simulink model "coalesce_walk_2d_sim"  (R2014b)
settings: Solver=ode45  StartTime=0.0  StopTime=t_end
InitFcn:
  | colors
  | simulation_params
  | mechanical_params
StartFcn:
  | tic
StopFcn:
  | stopscript
values from neighbouring files (symbols this model uses):
  b_hmotor = 0    [mechanical_params.m]
  b_leg_spring = 0.075*sqrt(k_leg_spring*0.5*.25^2)    [mechanical_params.m]
  b_rotor = 0*60/(2*pi)*9.725e-5    (= 0)    [mechanical_params.m]
  breakaway_friction = [25 25 25 25]    [mechanical_params.m]
  coulomb_friction = [20 20 20 20]    [mechanical_params.m]
  d_com = (d_hip_com_to_torso_com*m_torso)/(m_torso + num_legs*m_hshaft)    [mechanical_params.m]
  delta_phi_max = 160*pi/180    (= 2.79252680319)    [mechanical_params.m]
  delta_phi_min = 25.5*pi/180    (= 0.445058959259)    [mechanical_params.m]
  friction_linear_zone = [0.5 0.5 0.5 0.5].*pi/180    [mechanical_params.m]
  g = 9.81    [mechanical_params.m]
  HIP_MTR_MAX_TORQUE = max_current_hip*Kt_hip*N_h    (= 629.28)    [mechanical_params.m]
  initial_boom_pitch = 0    [mechanical_params.m]
  initial_boom_roll = asin((initial_com_height + boom_mount_to_com + boom_mount_to_center*tan(pitch_mount_angle) - (base_12(2) + yshaft_12(2))) / (l_boom + boom_mount_to_center_diagonal))    [mechanical_params.m]
  initial_boom_yaw = 0    [mechanical_params.m]
  initial_hip_roll = 0*pi/180    (= 0)    [mechanical_params.m]
  initial_winch_angle = -12 * pi/180    (= -0.209439510239)    [mechanical_params.m]
  k_gx = m_total*g/0.01    (= 57082.15332)    [mechanical_params.m]
  k_gy = m_total*g/0.005    (= 114164.30664)    [mechanical_params.m]
  k_leg_spring = 2950    [mechanical_params.m]
  k_phi = 5000    [mechanical_params.m]
  Kb_leg = 0.121    [mechanical_params.m]
  kd_winch = td_winch*kp_winch    (= 989.945961256)    [mechanical_params.m]
  kp_winch = winch_gravity_comp/(3*pi/180)    (= 19798.9192251)    [mechanical_params.m]
  Kt_leg = 0.121    [mechanical_params.m]
  L_leg = 0.102e-3    (= 0.000102)    [mechanical_params.m]
  l_seg = 0.5    [mechanical_params.m]
  LEG_MTR_MAX_TORQUE = max_current_leg * Kt_leg * N    (= 1210)    [mechanical_params.m]
  lowerleg_12 = 0.40    (= 0.4)    [mechanical_params.m]
  m_boom = 4.49    [mechanical_params.m]
  m_fblink = 0.46    [mechanical_params.m]
  m_hshaft = 18    [mechanical_params.m]
  m_lowerleg = 0.4438    [mechanical_params.m]
  m_output_gear = 1e-5    (= 1e-05)    [mechanical_params.m]
  m_rotor = 1e-5    (= 1e-05)    [mechanical_params.m]
  m_shin = 0.75    [mechanical_params.m]
  m_thigh = 0.69    [mechanical_params.m]
  m_torso = 17.5    [mechanical_params.m]
  m_total = num_legs*(m_hshaft + m_thigh + m_lowerleg + m_shin + m_fblink + 2*m_gearing) + m_torso    (= 58.18772)    [mechanical_params.m]
  m_virtual_gear = 1e-5    (= 1e-05)    [mechanical_params.m]
  m_yshaft = 12.89    [mechanical_params.m]
  max_current_leg = 200    [mechanical_params.m]
  max_voltage_leg = 50    [mechanical_params.m]
  mu_hmotor = 0.90    (= 0.9)    [mechanical_params.m]
  mu_motor = 0.85    [mechanical_params.m]
  mu_slide = 0.95    [mechanical_params.m]
  mu_stick = 1.00    (= 1)    [mechanical_params.m]
  N = 50    [mechanical_params.m]
  N_h = r_hip_shaft / r_hip_gearhead    (= 57)    [mechanical_params.m]
  phi_max_collision = -5*pi/180    (= -0.0872664625997)    [mechanical_params.m]
  phi_roll_max = pi + 16*pi/180    (= 3.42084533391)    [mechanical_params.m]
  phi_roll_min = pi - 9*pi/180    (= 2.98451302091)    [mechanical_params.m]
  phi_shin_max = 3*pi/2 + 17.5*pi/180    (= 5.01782159948)    [mechanical_params.m]
  phi_shin_min = pi - 45*pi/180    (= 2.35619449019)    [mechanical_params.m]
  phi_thigh_max = pi + 45*pi/180    (= 3.92699081699)    [mechanical_params.m]
  phi_thigh_min = pi/2 - 17.5*pi/180    (= 1.2653637077)    [mechanical_params.m]
  r_hip_gearhead = 0.009525    [mechanical_params.m]
  r_hip_shaft = 0.542925    [mechanical_params.m]
  R_leg = 0.052    [mechanical_params.m]
  r_rotor = 0.001    [mechanical_params.m]
  r_virtual_gear = N*r_rotor    (= 0.05)    [mechanical_params.m]
  s = clamp(s, 0, 1)    [controller.m]
  shin_12 = 0.40    (= 0.4)    [mechanical_params.m]
  shin_initial_l = initial_l_leg_angle + acos(initial_l_leg_length)    [mechanical_params.m]
  shin_initial_r = initial_r_leg_angle + acos(initial_r_leg_length)    [mechanical_params.m]
  thigh_initial_l = initial_l_leg_angle - acos(initial_l_leg_length)    [mechanical_params.m]
  thigh_initial_r = initial_r_leg_angle - acos(initial_r_leg_length)    [mechanical_params.m]
  tile_color = cmap(floor((tile_scale/(max_floor_tile_height+eps))*length(cmap))+1,:)    [mechanical_params.m]
  tile_cross_section = [1.5 0.03; 1.5 0; 3 0; 3 0.03]    [mechanical_params.m]
  tile_delta = [0 1; 0 0; 0 0; 0 1]    [mechanical_params.m]
  tile_scale = zeros(12, 1)    [mechanical_params.m]
  v_gx_max = 0.03    [mechanical_params.m]
  v_gy_max = 0.03    [mechanical_params.m]
  v_phi_max = 1/60    (= 0.0166666666667)    [mechanical_params.m]
  viscous_friction = [0.001 0.001 0.001 0.001]    [mechanical_params.m]
  vLimit = 0.01    [mechanical_params.m]
undefined symbols (not defined in the file or in its folder): A_lpf_velocity, B1_lpf_velocity, B2_lpf_velocity, base_color_d, boom_color_d, fblink_color_d, floor_color_d, hshaft_color_d, lowerleg_color_d, output_sample_time, rad, sample_time, sgn, shin_color_d, t_friction, thigh_color_d, torso_color_d, X, Y, yshaft_color_d, Z
libraries: sm_lib x196, nesl_utility x125, simulink x48, fl_lib x16, simulink_extras x2, mblibv1 x2, commnoisgen2 x1
(part 6 of 8)

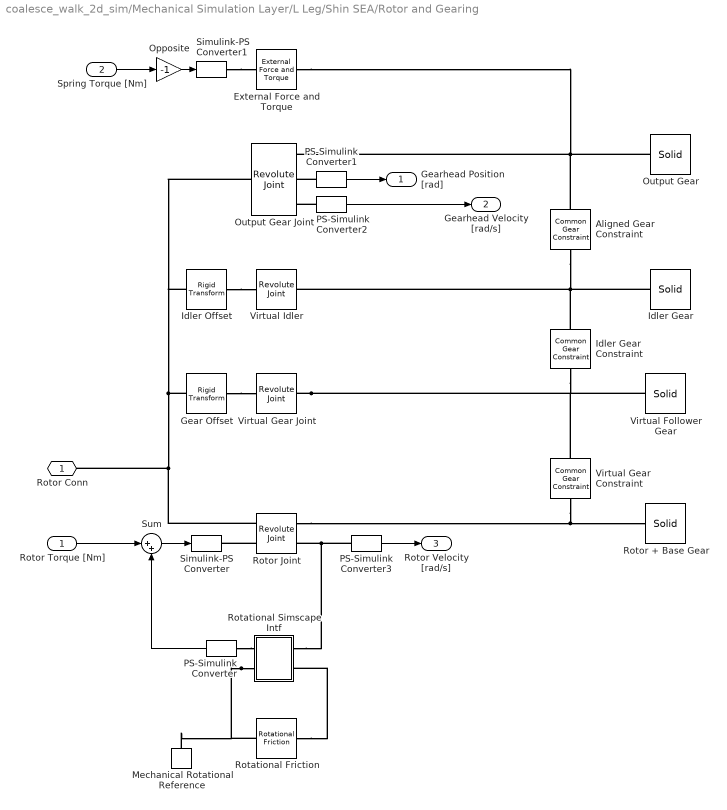
== system coalesce_walk_2d_sim/Mechanical Simulation Layer/L Leg/Shin SEA/Rotor and Gearing ==
  Rotor Torque [Nm] : Inport
  Spring Torque [Nm] : Inport  Port=2
  Aligned Gear Constraint : sm_lib/Gears and Couplings/Gears/Common Gear Constraint  GearType=External  SpecificationType=CenterDistanceRatio  CenterDistance=(r_rotor+r_virtual_gear)/2  CenterDistanceUnits=m  GearRatio=1  BaseGearRadius=1  BaseGearRadiusUnits=m  FollGearRadius=1  FollGearRadiusUnits=m  AssemblyGearRotation=Free  BlockFunction=simmechanics.library.gears_couplings_drives.gears.common_gear
  External Force and Torque : sm_lib/Forces and Torques/External Force and Torque  ForceResolutionFrame=AttachedFrame  EnableForceX=off  EnableForceY=off  EnableForceZ=off  EnableForce=off  TorqueResolutionFrame=AttachedFrame  EnableTorqueX=off  EnableTorqueY=off  EnableTorqueZ=on  EnableTorque=off  BlockFunction=simmechanics.library.forces_torques.external_force_torque
  Gear Offset : sm_lib/Frames and Transforms/Rigid Transform  TranslationMethod=Cartesian  TranslationLengthUnit=m  TranslationStandardAxis=+Z  TranslationStandardOffset=0  TranslationCartesianOffset=[(r_rotor+r_virtual_gear) 0 0]  TranslationROffset=0  TranslationROffsetUnits=m  TranslationZOffset=0  TranslationZOffsetUnits=m  TranslationThetaOffset=0  TranslationThetaOffsetUnits=deg  RotationMethod=None  RotationAngleUnits=deg  RotationStandardAxis=+Z  RotationAngle=0  RotationArbitraryAxis=[0 0 1]  FollAlignAxisA=+X  BaseAlignAxisA=+Y  FollAlignAxisB=+Y  BaseAlignAxisB=+Z  RotationMatrix=[1 0 0; 0 1 0; 0 0 1]  BlockFunction=simmechanics.library.frames_transforms.rigid_transform
  Idler Gear : sm_lib/Body Elements/Solid  InertiaType=Custom  Mass=m_virtual_gear  MassUnits=kg  CenterOfMass=[0 0 0]  CenterOfMassUnits=m  MomentsOfInertia=i_virtual_gear  MomentsOfInertiaUnits=kg*m^2  ProductsOfInertia=[0 0 0]  ProductsOfInertiaUnits=kg*m^2  DensityBased=on  Density=1000  DensityUnits=kg/(m^3)  GraphicType=None  MarkerShape=Sphere  MarkerSize=10  MarkerSizeUnits=m  GraphicVisPropType=SimpleVisualProperties  GraphicDiffuseColor=[1.0 0.2 0.2]  GraphicSpecularColor=[0.5 0.5 0.5 1.0]  GraphicAmbientColor=[0.15 0.15 0.15 1.0]  GraphicEmissiveColor=[0.0 0.0 0.0 1.0]  GraphicShininess=75  GraphicOpacity=1.0  GeometryShape=Cylinder  RectangleSize=[1 1]  RectangleSizeUnits=m  BrickDimensions=[1 1 1]  BrickDimensionUnits=m  CylinderRadius=r_virtual_gear  CylinderRadiusUnits=m  CylinderLength=0.01  CylinderLengthUnits=m  SphereRadius=1  SphereRadiusUnits=m  EllipsoidRadii=[1 1 1]  EllipsoidRadiiUnits=m  ExtrusionCrossSection=[1 1; -1 1; -1 -1; 1 -1]  ExtrusionCrossSectionUnits=m  ExtrusionLength=.2  ExtrusionLengthUnits=m  PolygonNumSides=3  PolygonOuterRadius=.3  PolygonOuterRadiusUnits=m  ExtGeomFileType=STL  ExtGeomFileUnits=m  RevolutionCrossSection=[1 1; 1 -1; 2 -1; 2 1]  RevolutionCrossSectionUnits=m  RevolutionExtent=Full  RevolutionAngle=180  RevolutionAngleUnits=deg  BlockFunction=simmechanics.library.body_elements.solid
  Idler Gear Constraint : sm_lib/Gears and Couplings/Gears/Common Gear Constraint  GearType=External  SpecificationType=CenterDistanceRatio  CenterDistance=(r_rotor+r_virtual_gear)/2  CenterDistanceUnits=m  GearRatio=1.0  BaseGearRadius=r_rotor  BaseGearRadiusUnits=m  FollGearRadius=r_virtual_gear  FollGearRadiusUnits=m  AssemblyGearRotation=Free  BlockFunction=simmechanics.library.gears_couplings_drives.gears.common_gear
  Idler Offset : sm_lib/Frames and Transforms/Rigid Transform  TranslationMethod=Cartesian  TranslationLengthUnit=m  TranslationStandardAxis=+Z  TranslationStandardOffset=0  TranslationCartesianOffset=[(r_rotor+r_virtual_gear)/2 0 0]  TranslationROffset=0  TranslationROffsetUnits=m  TranslationZOffset=0  TranslationZOffsetUnits=m  TranslationThetaOffset=0  TranslationThetaOffsetUnits=deg  RotationMethod=None  RotationAngleUnits=deg  RotationStandardAxis=+Z  RotationAngle=0  RotationArbitraryAxis=[0 0 1]  FollAlignAxisA=+X  BaseAlignAxisA=+Y  FollAlignAxisB=+Y  BaseAlignAxisB=+Z  RotationMatrix=[1 0 0; 0 1 0; 0 0 1]  BlockFunction=simmechanics.library.frames_transforms.rigid_transform
  Mechanical Rotational Reference : fl_lib/Mechanical/Rotational Elements/Mechanical Rotational Reference
  Opposite : Gain  Gain=-1
  Output Gear Joint : sm_lib/Joints/Revolute Joint  SenseConstraintForce=off  SenseConstraintForceX=off  SenseConstraintForceY=off  SenseConstraintForceZ=off  SenseConstraintTorque=off  SenseConstraintTorqueX=off  SenseConstraintTorqueY=off  SenseConstraintTorqueZ=off  SenseTotalForce=off  SenseTotalForceX=off  SenseTotalForceY=off  SenseTotalForceZ=off  SenseTotalTorque=off  SenseTotalTorqueX=off  SenseTotalTorqueY=off  SenseTotalTorqueZ=off  CompositeWrenchDir=FollowerOnBase  CompositeWrenchFrame=BaseFrame  EquilibriumPosition=0  EquilibriumPositionUnits=deg  SpringStiffness=0  SpringStiffnessUnits=N*m/deg  DampingCoefficient=0  DampingCoefficientUnits=N*m/(deg/s)  TorqueActuationMode=NoTorque  MotionActuationMode=ComputedMotion  SensePosition=on  SenseVelocity=on  SenseAcceleration=off  SenseTorqueForce=off  PositionTargetValue=0  PositionTargetValueUnits=deg  PositionTargetSpecify=off  PositionTargetPriority=High  VelocityTargetValue=0  VelocityTargetValueUnits=deg/s  VelocityTargetSpecify=off  VelocityTargetPriority=High  BlockFunction=simmechanics.library.joints.revolute_joint
  Output Gear : sm_lib/Body Elements/Solid  InertiaType=Custom  Mass=m_output_gear  MassUnits=kg  CenterOfMass=[0 0 0]  CenterOfMassUnits=m  MomentsOfInertia=i_output_gear  MomentsOfInertiaUnits=kg*m^2  ProductsOfInertia=[0 0 0]  ProductsOfInertiaUnits=kg*m^2  DensityBased=on  Density=1000  DensityUnits=kg/(m^3)  GraphicType=None  MarkerShape=Sphere  MarkerSize=10  MarkerSizeUnits=m  GraphicVisPropType=SimpleVisualProperties  GraphicDiffuseColor=[1.0 0.2 0.0]  GraphicSpecularColor=[0.5 0.5 0.5 1.0]  GraphicAmbientColor=[0.15 0.15 0.15 1.0]  GraphicEmissiveColor=[0.0 0.0 0.0 1.0]  GraphicShininess=75  GraphicOpacity=1.0  GeometryShape=Cylinder  RectangleSize=[1 1]  RectangleSizeUnits=m  BrickDimensions=[1 1 1]  BrickDimensionUnits=m  CylinderRadius=0.03  CylinderRadiusUnits=m  CylinderLength=0.01  CylinderLengthUnits=m  SphereRadius=1  SphereRadiusUnits=m  EllipsoidRadii=[1 1 1]  EllipsoidRadiiUnits=m  ExtrusionCrossSection=[1 1; -1 1; -1 -1; 1 -1]  ExtrusionCrossSectionUnits=m  ExtrusionLength=1  ExtrusionLengthUnits=m  PolygonNumSides=3  PolygonOuterRadius=1  PolygonOuterRadiusUnits=m  ExtGeomFileType=STL  ExtGeomFileUnits=m  RevolutionCrossSection=[1 1; 1 -1; 2 -1; 2 1]  RevolutionCrossSectionUnits=m  RevolutionExtent=Full  RevolutionAngle=180  RevolutionAngleUnits=deg  BlockFunction=simmechanics.library.body_elements.solid
  PS-Simulink Converter{,1..3} (4 alike) : nesl_utility/PS-Simulink Converter  PhysicalDomain=network_engine_domain  SubClassName=ps_output  LeftPortType=input  RightPortType=output  PseudoPeriodic=off  Frequencies=[]  Unit=1  AffineConversion=off
  Rotational Simscape Intf : Subsystem
  Rotational Friction : fl_lib/Mechanical/Rotational Elements/Rotational Friction  brkwy_trq=breakaway_friction(3)/N N*m  Col_trq=coulomb_friction(3)/N N*m  visc_coef=viscous_friction(3)/N N*m/(rad/s)  trans_coef=10 s/rad  vel_thr=friction_linear_zone(3)*N rad/s  w_specify=off  w_priority=High  w=0 rad/s  t_specify=off  t_priority=High  t=0 N*m
  Rotor + Base Gear : sm_lib/Body Elements/Solid  InertiaType=Custom  Mass=m_rotor  MassUnits=kg  CenterOfMass=[0 0 0]  CenterOfMassUnits=m  MomentsOfInertia=i_rotor_moments  MomentsOfInertiaUnits=kg*m^2  ProductsOfInertia=[0 0 0]  ProductsOfInertiaUnits=kg*m^2  DensityBased=on  Density=1000  DensityUnits=kg/(m^3)  GraphicType=None  MarkerShape=Sphere  MarkerSize=10  MarkerSizeUnits=m  GraphicVisPropType=AdvancedVisualProperties  GraphicDiffuseColor=[0.5 0.5 0.5]  GraphicSpecularColor=[0.5 0.5 0.5 1.0]  GraphicAmbientColor=[0.15 0.15 0.15 1.0]  GraphicEmissiveColor=[0.0 0.0 0.0 1.0]  GraphicShininess=10  GraphicOpacity=1.0  GeometryShape=Cylinder  RectangleSize=[1 1]  RectangleSizeUnits=m  BrickDimensions=[1 1 1]  BrickDimensionUnits=m  CylinderRadius=0.01  CylinderRadiusUnits=m  CylinderLength=0.01  CylinderLengthUnits=m  SphereRadius=1  SphereRadiusUnits=m  EllipsoidRadii=[1 1 1]  EllipsoidRadiiUnits=m  ExtrusionCrossSection=[1 1; -1 1; -1 -1; 1 -1]  ExtrusionCrossSectionUnits=m  ExtrusionLength=0.4  ExtrusionLengthUnits=m  PolygonNumSides=3  PolygonOuterRadius=0.2  PolygonOuterRadiusUnits=m  ExtGeomFileType=STL  ExtGeomFileUnits=m  RevolutionCrossSection=[1 1; 1 -1; 2 -1; 2 1]  RevolutionCrossSectionUnits=m  RevolutionExtent=Full  RevolutionAngle=180  RevolutionAngleUnits=deg  BlockFunction=simmechanics.library.body_elements.solid
  Rotor Joint : sm_lib/Joints/Revolute Joint  SenseConstraintForce=off  SenseConstraintForceX=off  SenseConstraintForceY=off  SenseConstraintForceZ=off  SenseConstraintTorque=off  SenseConstraintTorqueX=off  SenseConstraintTorqueY=off  SenseConstraintTorqueZ=off  SenseTotalForce=off  SenseTotalForceX=off  SenseTotalForceY=off  SenseTotalForceZ=off  SenseTotalTorque=off  SenseTotalTorqueX=off  SenseTotalTorqueY=off  SenseTotalTorqueZ=off  CompositeWrenchDir=FollowerOnBase  CompositeWrenchFrame=BaseFrame  EquilibriumPosition=0  EquilibriumPositionUnits=deg  SpringStiffness=0  SpringStiffnessUnits=N*m/deg  DampingCoefficient=0  DampingCoefficientUnits=N*m/(deg/s)  TorqueActuationMode=InputTorque  MotionActuationMode=ComputedMotion  SensePosition=off  SenseVelocity=on  SenseAcceleration=off  SenseTorqueForce=off  PositionTargetValue=0  PositionTargetValueUnits=deg  PositionTargetSpecify=off  PositionTargetPriority=High  VelocityTargetValue=0  VelocityTargetValueUnits=deg/s  VelocityTargetSpecify=off  VelocityTargetPriority=High  BlockFunction=simmechanics.library.joints.revolute_joint
  Simulink-PS Converter : nesl_utility/Simulink-PS Converter  PhysicalDomain=network_engine_domain  SubClassName=ps_input  LeftPortType=input  RightPortType=output  PseudoPeriodic=off  Frequencies=[]  NoiseDistribution=none  NoiseParameters=[]  Unit=1  AffineConversion=off  InputFiltering=off  SimscapeFilterOrder=1  InputFilterTimeConstant=0.001  UdotUserProvided=1
  Simulink-PS Converter1 : nesl_utility/Simulink-PS Converter  PhysicalDomain=network_engine_domain  SubClassName=ps_input  LeftPortType=input  RightPortType=output  PseudoPeriodic=off  Frequencies=[]  NoiseDistribution=none  NoiseParameters=[]  Unit=1  AffineConversion=off  InputFiltering=off  SimscapeFilterOrder=1  InputFilterTimeConstant=0.001  UdotUserProvided=1
  Sum : Sum  Inputs=|++
  Virtual Gear Joint : sm_lib/Joints/Revolute Joint  SenseConstraintForce=off  SenseConstraintForceX=off  SenseConstraintForceY=off  SenseConstraintForceZ=off  SenseConstraintTorque=off  SenseConstraintTorqueX=off  SenseConstraintTorqueY=off  SenseConstraintTorqueZ=off  SenseTotalForce=off  SenseTotalForceX=off  SenseTotalForceY=off  SenseTotalForceZ=off  SenseTotalTorque=off  SenseTotalTorqueX=off  SenseTotalTorqueY=off  SenseTotalTorqueZ=off  CompositeWrenchDir=FollowerOnBase  CompositeWrenchFrame=BaseFrame  EquilibriumPosition=0  EquilibriumPositionUnits=deg  SpringStiffness=0  SpringStiffnessUnits=N*m/deg  DampingCoefficient=0  DampingCoefficientUnits=N*m/(deg/s)  TorqueActuationMode=NoTorque  MotionActuationMode=ComputedMotion  SensePosition=off  SenseVelocity=off  SenseAcceleration=off  SenseTorqueForce=off  PositionTargetValue=0  PositionTargetValueUnits=deg  PositionTargetSpecify=off  PositionTargetPriority=High  VelocityTargetValue=0  VelocityTargetValueUnits=deg/s  VelocityTargetSpecify=off  VelocityTargetPriority=High  BlockFunction=simmechanics.library.joints.revolute_joint
  Virtual Follower Gear : sm_lib/Body Elements/Solid  InertiaType=Custom  Mass=m_virtual_gear  MassUnits=kg  CenterOfMass=[0 0 0]  CenterOfMassUnits=m  MomentsOfInertia=i_virtual_gear  MomentsOfInertiaUnits=kg*m^2  ProductsOfInertia=[0 0 0]  ProductsOfInertiaUnits=kg*m^2  DensityBased=on  Density=1000  DensityUnits=kg/(m^3)  GraphicType=None  MarkerShape=Sphere  MarkerSize=10  MarkerSizeUnits=m  GraphicVisPropType=SimpleVisualProperties  GraphicDiffuseColor=[1.0 0.2 0.2]  GraphicSpecularColor=[0.5 0.5 0.5 1.0]  GraphicAmbientColor=[0.15 0.15 0.15 1.0]  GraphicEmissiveColor=[0.0 0.0 0.0 1.0]  GraphicShininess=75  GraphicOpacity=1.0  GeometryShape=Cylinder  RectangleSize=[1 1]  RectangleSizeUnits=m  BrickDimensions=[1 1 1]  BrickDimensionUnits=m  CylinderRadius=r_virtual_gear  CylinderRadiusUnits=m  CylinderLength=0.01  CylinderLengthUnits=m  SphereRadius=1  SphereRadiusUnits=m  EllipsoidRadii=[1 1 1]  EllipsoidRadiiUnits=m  ExtrusionCrossSection=[1 1; -1 1; -1 -1; 1 -1]  ExtrusionCrossSectionUnits=m  ExtrusionLength=.2  ExtrusionLengthUnits=m  PolygonNumSides=3  PolygonOuterRadius=.3  PolygonOuterRadiusUnits=m  ExtGeomFileType=STL  ExtGeomFileUnits=m  RevolutionCrossSection=[1 1; 1 -1; 2 -1; 2 1]  RevolutionCrossSectionUnits=m  RevolutionExtent=Full  RevolutionAngle=180  RevolutionAngleUnits=deg  BlockFunction=simmechanics.library.body_elements.solid
  Virtual Gear Constraint : sm_lib/Gears and Couplings/Gears/Common Gear Constraint  GearType=External  SpecificationType=PitchCircleRadii  CenterDistance=20.0  CenterDistanceUnits=cm  GearRatio=1.0  BaseGearRadius=r_rotor  BaseGearRadiusUnits=m  FollGearRadius=r_virtual_gear  FollGearRadiusUnits=m  AssemblyGearRotation=Free  BlockFunction=simmechanics.library.gears_couplings_drives.gears.common_gear
  Virtual Idler : sm_lib/Joints/Revolute Joint  SenseConstraintForce=off  SenseConstraintForceX=off  SenseConstraintForceY=off  SenseConstraintForceZ=off  SenseConstraintTorque=off  SenseConstraintTorqueX=off  SenseConstraintTorqueY=off  SenseConstraintTorqueZ=off  SenseTotalForce=off  SenseTotalForceX=off  SenseTotalForceY=off  SenseTotalForceZ=off  SenseTotalTorque=off  SenseTotalTorqueX=off  SenseTotalTorqueY=off  SenseTotalTorqueZ=off  CompositeWrenchDir=FollowerOnBase  CompositeWrenchFrame=BaseFrame  EquilibriumPosition=0  EquilibriumPositionUnits=deg  SpringStiffness=0  SpringStiffnessUnits=N*m/deg  DampingCoefficient=0  DampingCoefficientUnits=N*m/(deg/s)  TorqueActuationMode=NoTorque  MotionActuationMode=ComputedMotion  SensePosition=off  SenseVelocity=off  SenseAcceleration=off  SenseTorqueForce=off  PositionTargetValue=0  PositionTargetValueUnits=deg  PositionTargetSpecify=off  PositionTargetPriority=High  VelocityTargetValue=0  VelocityTargetValueUnits=deg/s  VelocityTargetSpecify=off  VelocityTargetPriority=High  BlockFunction=simmechanics.library.joints.revolute_joint
  Rotor Conn : PMIOPort  Port=1  Side=Left
  Gearhead Position [rad] : Outport
  Gearhead Velocity [rad/s] : Outport  Port=2
  Rotor Velocity [rad/s] : Outport  Port=3
  wires:
  PS-Simulink Converter1/1 -> Gearhead Position [rad]/1
  Rotor Torque [Nm]/1 -> Sum/1
  PS-Simulink Converter2/1 -> Gearhead Velocity [rad/s]/1
  PS-Simulink Converter3/1 -> Rotor Velocity [rad/s]/1
  Spring Torque [Nm]/1 -> Opposite/1
  Opposite/1 -> Simulink-PS Converter1/1
  PS-Simulink Converter/1 -> Sum/2
  Sum/1 -> Simulink-PS Converter/1
  connections:
  Virtual Gear Joint/RConn1 -- Virtual Follower Gear/RConn1 -- Virtual Gear Constraint/RConn1 -- Idler Gear Constraint/LConn1
  External Force and Torque/RConn1 -- Output Gear/RConn1 -- Aligned Gear Constraint/RConn1 -- Output Gear Joint/RConn1
  Gear Offset/RConn1 -- Virtual Gear Joint/LConn1
  Gear Offset/LConn1 -- Rotor Joint/LConn1 -- Rotor Conn/RConn1 -- Output Gear Joint/LConn1 -- Idler Offset/LConn1
  Rotor Joint/RConn1 -- Virtual Gear Constraint/LConn1 -- Rotor + Base Gear/RConn1
  Rotor Joint/LConn2 -- Simulink-PS Converter/RConn1
  PS-Simulink Converter2/LConn1 -- Output Gear Joint/RConn3
  PS-Simulink Converter1/LConn1 -- Output Gear Joint/RConn2
  PS-Simulink Converter3/LConn1 -- Rotational Simscape Intf/LConn1 -- Rotor Joint/RConn2
  Simulink-PS Converter1/RConn1 -- External Force and Torque/LConn1
  Idler Gear Constraint/RConn1 -- Virtual Idler/RConn1 -- Idler Gear/RConn1 -- Aligned Gear Constraint/LConn1
  Idler Offset/RConn1 -- Virtual Idler/LConn1
  Rotational Simscape Intf/RConn2 -- Mechanical Rotational Reference/LConn1 -- Rotational Friction/RConn1
  Rotational Friction/LConn1 -- Rotational Simscape Intf/LConn2
  PS-Simulink Converter/LConn1 -- Rotational Simscape Intf/RConn1

== system coalesce_walk_2d_sim/Mechanical Simulation Layer/L Leg/Thigh/Frame Data ==
  Kinematic Data : ToWorkspace  VariableName=l_thigh_out  SampleTime=output_sample_time
      settings: Save2DSignal=2-D array (concatenate along first dimension)
  Mux : Mux
  PS-Simulink Converter{,1..3} (4 alike) : nesl_utility/PS-Simulink Converter  PhysicalDomain=network_engine_domain  SubClassName=ps_output  LeftPortType=input  RightPortType=output  PseudoPeriodic=off  Frequencies=[]  Unit=1  AffineConversion=off
  Transform Sensor : sm_lib/Frames and Transforms/Transform Sensor  MeasurementFrame=World  SenseAngle=off  SenseAxis=off  SenseAngle1=off  SenseAngle2=off  SenseAngle3=off  SenseQ=on  SenseR=off  SenseOmegaX=off  SenseOmegaY=off  SenseOmegaZ=off  SenseOmega1=off  SenseOmega2=off  SenseOmega3=off  SenseQDot=off  SenseRDot=off  SenseAlphaX=off  SenseAlphaY=off  SenseAlphaZ=off  SenseAlpha1=off  SenseAlpha2=off  SenseAlpha3=off  SenseQDDot=off  SenseRDDot=off  SenseX=on  SenseY=on  SenseZ=on  SenseRad=off  SenseAzim=off  SenseDist=off  SenseInc=off  SenseXDot=off  SenseYDot=off  SenseZDot=off  SenseRadDot=off  SenseAzimDot=off  SenseDistDot=off  SenseIncDot=off  SenseXDDot=off  SenseYDDot=off  SenseZDDot=off  SenseRadDDot=off  SenseAzimDDot=off  SenseDistDDot=off  SenseIncDDot=off  BlockFunction=simmechanics.library.frames_transforms.transform_sensor
  World Frame : sm_lib/Frames and Transforms/World Frame  BlockFunction=simmechanics.library.frames_transforms.world_frame
  Frame : PMIOPort  Port=1  Side=Left
  wires:
  Mux/1 -> Kinematic Data/1
  PS-Simulink Converter/1 -> Mux/1
  PS-Simulink Converter1/1 -> Mux/2
  PS-Simulink Converter2/1 -> Mux/3
  PS-Simulink Converter3/1 -> Mux/4
  connections:
  PS-Simulink Converter3/LConn1 -- Transform Sensor/RConn5
  PS-Simulink Converter2/LConn1 -- Transform Sensor/RConn4
  PS-Simulink Converter1/LConn1 -- Transform Sensor/RConn3
  PS-Simulink Converter/LConn1 -- Transform Sensor/RConn2
  Transform Sensor/RConn1 -- Frame/RConn1
  Transform Sensor/LConn1 -- World Frame/RConn1

== system coalesce_walk_2d_sim/Mechanical Simulation Layer/L Leg/Thigh SEA/Motor Controller ==
  Desired Current [A] : Inport
  Measured Current [A] : Inport  Port=2
  Speed [rad/s] : Inport  Port=3
  Ke : Gain  Gain=Kb_leg
  PI Controller : simulink/Continuous/PID Controller  Controller=PI  TimeDomain=Continuous-time  SampleTime=-1  IntegratorMethod=Trapezoidal  FilterMethod=Forward Euler  Form=Parallel  P=0.57  I=0.016  D=0.016  N=10  InitialConditionSource=internal  InitialConditionForIntegrator=0  InitialConditionForFilter=0  ExternalReset=none  ZeroCross=off  LimitOutput=off  UpperSaturationLimit=inf  LowerSaturationLimit=-inf  LinearizeAsGain=on  AntiWindupMode=none  Kb=1  TrackingMode=off  Kt=1  PParamMin=[]  PParamMax=[]  IParamMin=[]  IParamMax=[]  DParamMin=[]  DParamMax=[]  NParamMin=[]  NParamMax=[]  KbParamMin=[]  KbParamMax=[]  KtParamMin=[]  KtParamMax=[]  POutMin=[]  POutMax=[]  IOutMin=[]  IOutMax=[]  DOutMin=[]  DOutMax=[]  NOutMin=[]  NOutMax=[]  KbOutMin=[]  KbOutMax=[]  KtOutMin=[]  KtOutMax=[]  IntegratorOutMin=[]  IntegratorOutMax=[]  FilterOutMin=[]  FilterOutMax=[]  SumOutMin=[]  SumOutMax=[]  SumI1OutMin=[]  SumI1OutMax=[]  SumI2OutMin=[]  SumI2OutMax=[]  SumI3OutMin=[]  SumI3OutMax=[]  SumDOutMin=[]  SumDOutMax=[]  SaturationOutMin=[]  SaturationOutMax=[]  IntegratorContinuousStateAttributes=''  IntegratorStateMustResolveToSignalObject=off  IntegratorRTWStateStorageClass=Auto  FilterContinuousStateAttributes=''  FilterStateMustResolveToSignalObject=off  FilterRTWStateStorageClass=Auto  DifferentiatorICPrevScaledInput=0  DifferentiatorOutMin=[]  DifferentiatorOutMax=[]  UseFilter=on
  Resistance : Gain  Gain=R_leg
  Sum : Sum  Inputs=|+-
  Sum1 : Sum  Inputs=|++
  Sum2 : Sum  Inputs=+|+
  Voltage [V] : Outport
  wires:
  Desired Current [A]/1 -> Sum/1
  Measured Current [A]/1 -> Resistance/1, Sum/2
  Sum/1 -> PI Controller/1
  PI Controller/1 -> Sum1/1
  Speed [rad/s]/1 -> Ke/1
  Sum2/1 -> Sum1/2
  Resistance/1 -> Sum2/1
  Ke/1 -> Sum2/2
  Sum1/1 -> Voltage [V]/1

== system coalesce_walk_2d_sim/Mechanical Simulation Layer/L Leg/Thigh SEA/Motor Electromagnetism ==
  Voltage [V] : Inport
  Speed [rad/s] : Inport  Port=2
  Add : Sum  Inputs=-+-
  Inductance : Gain  Gain=1/L_leg
  Integrator : Integrator  ZeroCross=off
  Ke : Gain  Gain=Kb_leg
  Resistance : Gain  Gain=R_leg
  Torque Limiter (outside) 1 : Saturate  UpperLimit=max_voltage_leg  LowerLimit=-max_voltage_leg  ZeroCross=off
      settings: AttributesFormatString=Hi: %<UpperLimit>\nLo: %<LowerLimit>
  Torque Limiter (outside) 2 : Saturate  UpperLimit=max_current_leg  LowerLimit=-max_current_leg  ZeroCross=off
      settings: AttributesFormatString=Hi: %<UpperLimit>\nLo: %<LowerLimit>
  Current [A] : Outport
  wires:
  Integrator/1 -> Torque Limiter (outside) 2/1  "I"
  Inductance/1 -> Integrator/1  "d/dt(I)"
  Speed [rad/s]/1 -> Ke/1  "d/dt(theta)"
  Add/1 -> Inductance/1
  Resistance/1 -> Add/1
  Ke/1 -> Add/3
  Voltage [V]/1 -> Torque Limiter (outside) 1/1
  Torque Limiter (outside) 2/1 -> Current [A]/1, Resistance/1
  Torque Limiter (outside) 1/1 -> Add/2

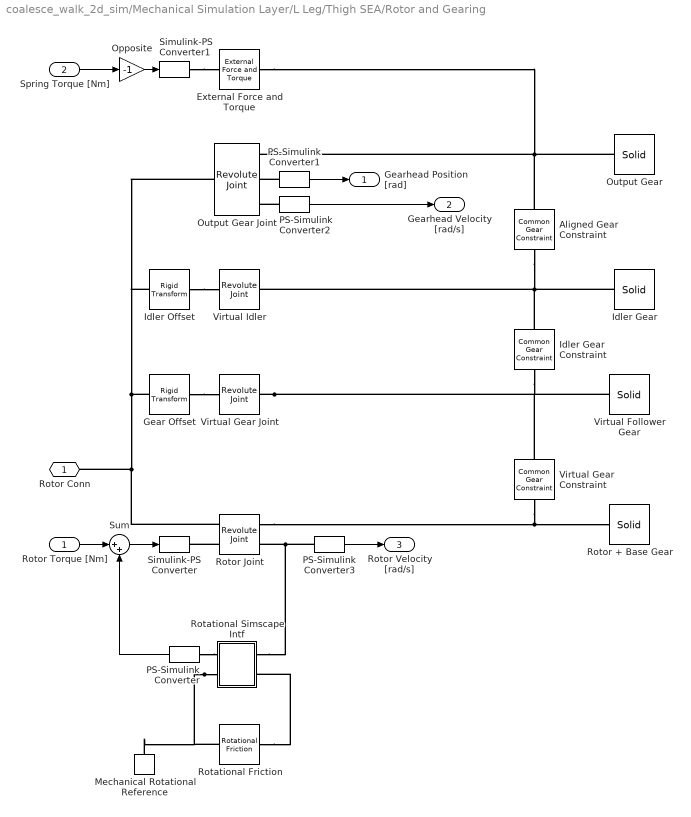
== system coalesce_walk_2d_sim/Mechanical Simulation Layer/L Leg/Thigh SEA/Rotor and Gearing ==
  Rotor Torque [Nm] : Inport
  Spring Torque [Nm] : Inport  Port=2
  Aligned Gear Constraint : sm_lib/Gears and Couplings/Gears/Common Gear Constraint  GearType=External  SpecificationType=CenterDistanceRatio  CenterDistance=(r_rotor+r_virtual_gear)/2  CenterDistanceUnits=m  GearRatio=1  BaseGearRadius=1  BaseGearRadiusUnits=m  FollGearRadius=1  FollGearRadiusUnits=m  AssemblyGearRotation=Free  BlockFunction=simmechanics.library.gears_couplings_drives.gears.common_gear
  External Force and Torque : sm_lib/Forces and Torques/External Force and Torque  ForceResolutionFrame=AttachedFrame  EnableForceX=off  EnableForceY=off  EnableForceZ=off  EnableForce=off  TorqueResolutionFrame=AttachedFrame  EnableTorqueX=off  EnableTorqueY=off  EnableTorqueZ=on  EnableTorque=off  BlockFunction=simmechanics.library.forces_torques.external_force_torque
  Gear Offset : sm_lib/Frames and Transforms/Rigid Transform  TranslationMethod=Cartesian  TranslationLengthUnit=m  TranslationStandardAxis=+Z  TranslationStandardOffset=0  TranslationCartesianOffset=[(r_rotor+r_virtual_gear) 0 0]  TranslationROffset=0  TranslationROffsetUnits=m  TranslationZOffset=0  TranslationZOffsetUnits=m  TranslationThetaOffset=0  TranslationThetaOffsetUnits=deg  RotationMethod=None  RotationAngleUnits=deg  RotationStandardAxis=+Z  RotationAngle=0  RotationArbitraryAxis=[0 0 1]  FollAlignAxisA=+X  BaseAlignAxisA=+Y  FollAlignAxisB=+Y  BaseAlignAxisB=+Z  RotationMatrix=[1 0 0; 0 1 0; 0 0 1]  BlockFunction=simmechanics.library.frames_transforms.rigid_transform
  Idler Gear : sm_lib/Body Elements/Solid  InertiaType=Custom  Mass=m_virtual_gear  MassUnits=kg  CenterOfMass=[0 0 0]  CenterOfMassUnits=m  MomentsOfInertia=i_virtual_gear  MomentsOfInertiaUnits=kg*m^2  ProductsOfInertia=[0 0 0]  ProductsOfInertiaUnits=kg*m^2  DensityBased=on  Density=1000  DensityUnits=kg/(m^3)  GraphicType=None  MarkerShape=Sphere  MarkerSize=10  MarkerSizeUnits=m  GraphicVisPropType=SimpleVisualProperties  GraphicDiffuseColor=[1.0 0.2 0.2]  GraphicSpecularColor=[0.5 0.5 0.5 1.0]  GraphicAmbientColor=[0.15 0.15 0.15 1.0]  GraphicEmissiveColor=[0.0 0.0 0.0 1.0]  GraphicShininess=75  GraphicOpacity=1.0  GeometryShape=Cylinder  RectangleSize=[1 1]  RectangleSizeUnits=m  BrickDimensions=[1 1 1]  BrickDimensionUnits=m  CylinderRadius=r_virtual_gear  CylinderRadiusUnits=m  CylinderLength=0.01  CylinderLengthUnits=m  SphereRadius=1  SphereRadiusUnits=m  EllipsoidRadii=[1 1 1]  EllipsoidRadiiUnits=m  ExtrusionCrossSection=[1 1; -1 1; -1 -1; 1 -1]  ExtrusionCrossSectionUnits=m  ExtrusionLength=.2  ExtrusionLengthUnits=m  PolygonNumSides=3  PolygonOuterRadius=.3  PolygonOuterRadiusUnits=m  ExtGeomFileType=STL  ExtGeomFileUnits=m  RevolutionCrossSection=[1 1; 1 -1; 2 -1; 2 1]  RevolutionCrossSectionUnits=m  RevolutionExtent=Full  RevolutionAngle=180  RevolutionAngleUnits=deg  BlockFunction=simmechanics.library.body_elements.solid
  Idler Gear Constraint : sm_lib/Gears and Couplings/Gears/Common Gear Constraint  GearType=External  SpecificationType=CenterDistanceRatio  CenterDistance=(r_rotor+r_virtual_gear)/2  CenterDistanceUnits=m  GearRatio=1.0  BaseGearRadius=r_rotor  BaseGearRadiusUnits=m  FollGearRadius=r_virtual_gear  FollGearRadiusUnits=m  AssemblyGearRotation=Free  BlockFunction=simmechanics.library.gears_couplings_drives.gears.common_gear
  Idler Offset : sm_lib/Frames and Transforms/Rigid Transform  TranslationMethod=Cartesian  TranslationLengthUnit=m  TranslationStandardAxis=+Z  TranslationStandardOffset=0  TranslationCartesianOffset=[(r_rotor+r_virtual_gear)/2 0 0]  TranslationROffset=0  TranslationROffsetUnits=m  TranslationZOffset=0  TranslationZOffsetUnits=m  TranslationThetaOffset=0  TranslationThetaOffsetUnits=deg  RotationMethod=None  RotationAngleUnits=deg  RotationStandardAxis=+Z  RotationAngle=0  RotationArbitraryAxis=[0 0 1]  FollAlignAxisA=+X  BaseAlignAxisA=+Y  FollAlignAxisB=+Y  BaseAlignAxisB=+Z  RotationMatrix=[1 0 0; 0 1 0; 0 0 1]  BlockFunction=simmechanics.library.frames_transforms.rigid_transform
  Mechanical Rotational Reference : fl_lib/Mechanical/Rotational Elements/Mechanical Rotational Reference
  Opposite : Gain  Gain=-1
  Output Gear Joint : sm_lib/Joints/Revolute Joint  SenseConstraintForce=off  SenseConstraintForceX=off  SenseConstraintForceY=off  SenseConstraintForceZ=off  SenseConstraintTorque=off  SenseConstraintTorqueX=off  SenseConstraintTorqueY=off  SenseConstraintTorqueZ=off  SenseTotalForce=off  SenseTotalForceX=off  SenseTotalForceY=off  SenseTotalForceZ=off  SenseTotalTorque=off  SenseTotalTorqueX=off  SenseTotalTorqueY=off  SenseTotalTorqueZ=off  CompositeWrenchDir=FollowerOnBase  CompositeWrenchFrame=BaseFrame  EquilibriumPosition=0  EquilibriumPositionUnits=deg  SpringStiffness=0  SpringStiffnessUnits=N*m/deg  DampingCoefficient=0  DampingCoefficientUnits=N*m/(deg/s)  TorqueActuationMode=NoTorque  MotionActuationMode=ComputedMotion  SensePosition=on  SenseVelocity=on  SenseAcceleration=off  SenseTorqueForce=off  PositionTargetValue=0  PositionTargetValueUnits=deg  PositionTargetSpecify=off  PositionTargetPriority=High  VelocityTargetValue=0  VelocityTargetValueUnits=deg/s  VelocityTargetSpecify=off  VelocityTargetPriority=High  BlockFunction=simmechanics.library.joints.revolute_joint
  Output Gear : sm_lib/Body Elements/Solid  InertiaType=Custom  Mass=m_output_gear  MassUnits=kg  CenterOfMass=[0 0 0]  CenterOfMassUnits=m  MomentsOfInertia=i_output_gear  MomentsOfInertiaUnits=kg*m^2  ProductsOfInertia=[0 0 0]  ProductsOfInertiaUnits=kg*m^2  DensityBased=on  Density=1000  DensityUnits=kg/(m^3)  GraphicType=None  MarkerShape=Sphere  MarkerSize=10  MarkerSizeUnits=m  GraphicVisPropType=SimpleVisualProperties  GraphicDiffuseColor=[1.0 0.2 0.0]  GraphicSpecularColor=[0.5 0.5 0.5 1.0]  GraphicAmbientColor=[0.15 0.15 0.15 1.0]  GraphicEmissiveColor=[0.0 0.0 0.0 1.0]  GraphicShininess=75  GraphicOpacity=1.0  GeometryShape=Cylinder  RectangleSize=[1 1]  RectangleSizeUnits=m  BrickDimensions=[1 1 1]  BrickDimensionUnits=m  CylinderRadius=0.03  CylinderRadiusUnits=m  CylinderLength=0.01  CylinderLengthUnits=m  SphereRadius=1  SphereRadiusUnits=m  EllipsoidRadii=[1 1 1]  EllipsoidRadiiUnits=m  ExtrusionCrossSection=[1 1; -1 1; -1 -1; 1 -1]  ExtrusionCrossSectionUnits=m  ExtrusionLength=1  ExtrusionLengthUnits=m  PolygonNumSides=3  PolygonOuterRadius=1  PolygonOuterRadiusUnits=m  ExtGeomFileType=STL  ExtGeomFileUnits=m  RevolutionCrossSection=[1 1; 1 -1; 2 -1; 2 1]  RevolutionCrossSectionUnits=m  RevolutionExtent=Full  RevolutionAngle=180  RevolutionAngleUnits=deg  BlockFunction=simmechanics.library.body_elements.solid
  PS-Simulink Converter{,1..3} (4 alike) : nesl_utility/PS-Simulink Converter  PhysicalDomain=network_engine_domain  SubClassName=ps_output  LeftPortType=input  RightPortType=output  PseudoPeriodic=off  Frequencies=[]  Unit=1  AffineConversion=off
  Rotational Simscape Intf : Subsystem
  Rotational Friction : fl_lib/Mechanical/Rotational Elements/Rotational Friction  brkwy_trq=breakaway_friction(4)/N N*m  Col_trq=coulomb_friction(4)/N N*m  visc_coef=viscous_friction(4)/N N*m/(rad/s)  trans_coef=10 s/rad  vel_thr=friction_linear_zone(4)*N rad/s  w_specify=off  w_priority=High  w=0 rad/s  t_specify=off  t_priority=High  t=0 N*m
  Rotor + Base Gear : sm_lib/Body Elements/Solid  InertiaType=Custom  Mass=m_rotor  MassUnits=kg  CenterOfMass=[0 0 0]  CenterOfMassUnits=m  MomentsOfInertia=i_rotor_moments  MomentsOfInertiaUnits=kg*m^2  ProductsOfInertia=[0 0 0]  ProductsOfInertiaUnits=kg*m^2  DensityBased=on  Density=1000  DensityUnits=kg/(m^3)  GraphicType=None  MarkerShape=Sphere  MarkerSize=10  MarkerSizeUnits=m  GraphicVisPropType=AdvancedVisualProperties  GraphicDiffuseColor=[0.5 0.5 0.5]  GraphicSpecularColor=[0.5 0.5 0.5 1.0]  GraphicAmbientColor=[0.15 0.15 0.15 1.0]  GraphicEmissiveColor=[0.0 0.0 0.0 1.0]  GraphicShininess=10  GraphicOpacity=1.0  GeometryShape=Cylinder  RectangleSize=[1 1]  RectangleSizeUnits=m  BrickDimensions=[1 1 1]  BrickDimensionUnits=m  CylinderRadius=0.01  CylinderRadiusUnits=m  CylinderLength=0.01  CylinderLengthUnits=m  SphereRadius=1  SphereRadiusUnits=m  EllipsoidRadii=[1 1 1]  EllipsoidRadiiUnits=m  ExtrusionCrossSection=[1 1; -1 1; -1 -1; 1 -1]  ExtrusionCrossSectionUnits=m  ExtrusionLength=0.4  ExtrusionLengthUnits=m  PolygonNumSides=3  PolygonOuterRadius=0.2  PolygonOuterRadiusUnits=m  ExtGeomFileType=STL  ExtGeomFileUnits=m  RevolutionCrossSection=[1 1; 1 -1; 2 -1; 2 1]  RevolutionCrossSectionUnits=m  RevolutionExtent=Full  RevolutionAngle=180  RevolutionAngleUnits=deg  BlockFunction=simmechanics.library.body_elements.solid
  Rotor Joint : sm_lib/Joints/Revolute Joint  SenseConstraintForce=off  SenseConstraintForceX=off  SenseConstraintForceY=off  SenseConstraintForceZ=off  SenseConstraintTorque=off  SenseConstraintTorqueX=off  SenseConstraintTorqueY=off  SenseConstraintTorqueZ=off  SenseTotalForce=off  SenseTotalForceX=off  SenseTotalForceY=off  SenseTotalForceZ=off  SenseTotalTorque=off  SenseTotalTorqueX=off  SenseTotalTorqueY=off  SenseTotalTorqueZ=off  CompositeWrenchDir=FollowerOnBase  CompositeWrenchFrame=BaseFrame  EquilibriumPosition=0  EquilibriumPositionUnits=deg  SpringStiffness=0  SpringStiffnessUnits=N*m/deg  DampingCoefficient=0  DampingCoefficientUnits=N*m/(deg/s)  TorqueActuationMode=InputTorque  MotionActuationMode=ComputedMotion  SensePosition=off  SenseVelocity=on  SenseAcceleration=off  SenseTorqueForce=off  PositionTargetValue=0  PositionTargetValueUnits=deg  PositionTargetSpecify=off  PositionTargetPriority=High  VelocityTargetValue=0  VelocityTargetValueUnits=deg/s  VelocityTargetSpecify=off  VelocityTargetPriority=High  BlockFunction=simmechanics.library.joints.revolute_joint
  Simulink-PS Converter : nesl_utility/Simulink-PS Converter  PhysicalDomain=network_engine_domain  SubClassName=ps_input  LeftPortType=input  RightPortType=output  PseudoPeriodic=off  Frequencies=[]  NoiseDistribution=none  NoiseParameters=[]  Unit=1  AffineConversion=off  InputFiltering=off  SimscapeFilterOrder=1  InputFilterTimeConstant=0.001  UdotUserProvided=1
  Simulink-PS Converter1 : nesl_utility/Simulink-PS Converter  PhysicalDomain=network_engine_domain  SubClassName=ps_input  LeftPortType=input  RightPortType=output  PseudoPeriodic=off  Frequencies=[]  NoiseDistribution=none  NoiseParameters=[]  Unit=1  AffineConversion=off  InputFiltering=off  SimscapeFilterOrder=1  InputFilterTimeConstant=0.001  UdotUserProvided=1
  Sum : Sum  Inputs=|++
  Virtual Gear Joint : sm_lib/Joints/Revolute Joint  SenseConstraintForce=off  SenseConstraintForceX=off  SenseConstraintForceY=off  SenseConstraintForceZ=off  SenseConstraintTorque=off  SenseConstraintTorqueX=off  SenseConstraintTorqueY=off  SenseConstraintTorqueZ=off  SenseTotalForce=off  SenseTotalForceX=off  SenseTotalForceY=off  SenseTotalForceZ=off  SenseTotalTorque=off  SenseTotalTorqueX=off  SenseTotalTorqueY=off  SenseTotalTorqueZ=off  CompositeWrenchDir=FollowerOnBase  CompositeWrenchFrame=BaseFrame  EquilibriumPosition=0  EquilibriumPositionUnits=deg  SpringStiffness=0  SpringStiffnessUnits=N*m/deg  DampingCoefficient=0  DampingCoefficientUnits=N*m/(deg/s)  TorqueActuationMode=NoTorque  MotionActuationMode=ComputedMotion  SensePosition=off  SenseVelocity=off  SenseAcceleration=off  SenseTorqueForce=off  PositionTargetValue=0  PositionTargetValueUnits=deg  PositionTargetSpecify=off  PositionTargetPriority=High  VelocityTargetValue=0  VelocityTargetValueUnits=deg/s  VelocityTargetSpecify=off  VelocityTargetPriority=High  BlockFunction=simmechanics.library.joints.revolute_joint
  Virtual Follower Gear : sm_lib/Body Elements/Solid  InertiaType=Custom  Mass=m_virtual_gear  MassUnits=kg  CenterOfMass=[0 0 0]  CenterOfMassUnits=m  MomentsOfInertia=i_virtual_gear  MomentsOfInertiaUnits=kg*m^2  ProductsOfInertia=[0 0 0]  ProductsOfInertiaUnits=kg*m^2  DensityBased=on  Density=1000  DensityUnits=kg/(m^3)  GraphicType=None  MarkerShape=Sphere  MarkerSize=10  MarkerSizeUnits=m  GraphicVisPropType=SimpleVisualProperties  GraphicDiffuseColor=[1.0 0.2 0.2]  GraphicSpecularColor=[0.5 0.5 0.5 1.0]  GraphicAmbientColor=[0.15 0.15 0.15 1.0]  GraphicEmissiveColor=[0.0 0.0 0.0 1.0]  GraphicShininess=75  GraphicOpacity=1.0  GeometryShape=Cylinder  RectangleSize=[1 1]  RectangleSizeUnits=m  BrickDimensions=[1 1 1]  BrickDimensionUnits=m  CylinderRadius=r_virtual_gear  CylinderRadiusUnits=m  CylinderLength=0.01  CylinderLengthUnits=m  SphereRadius=1  SphereRadiusUnits=m  EllipsoidRadii=[1 1 1]  EllipsoidRadiiUnits=m  ExtrusionCrossSection=[1 1; -1 1; -1 -1; 1 -1]  ExtrusionCrossSectionUnits=m  ExtrusionLength=.2  ExtrusionLengthUnits=m  PolygonNumSides=3  PolygonOuterRadius=.3  PolygonOuterRadiusUnits=m  ExtGeomFileType=STL  ExtGeomFileUnits=m  RevolutionCrossSection=[1 1; 1 -1; 2 -1; 2 1]  RevolutionCrossSectionUnits=m  RevolutionExtent=Full  RevolutionAngle=180  RevolutionAngleUnits=deg  BlockFunction=simmechanics.library.body_elements.solid
  Virtual Gear Constraint : sm_lib/Gears and Couplings/Gears/Common Gear Constraint  GearType=External  SpecificationType=PitchCircleRadii  CenterDistance=20.0  CenterDistanceUnits=cm  GearRatio=1.0  BaseGearRadius=r_rotor  BaseGearRadiusUnits=m  FollGearRadius=r_virtual_gear  FollGearRadiusUnits=m  AssemblyGearRotation=Free  BlockFunction=simmechanics.library.gears_couplings_drives.gears.common_gear
  Virtual Idler : sm_lib/Joints/Revolute Joint  SenseConstraintForce=off  SenseConstraintForceX=off  SenseConstraintForceY=off  SenseConstraintForceZ=off  SenseConstraintTorque=off  SenseConstraintTorqueX=off  SenseConstraintTorqueY=off  SenseConstraintTorqueZ=off  SenseTotalForce=off  SenseTotalForceX=off  SenseTotalForceY=off  SenseTotalForceZ=off  SenseTotalTorque=off  SenseTotalTorqueX=off  SenseTotalTorqueY=off  SenseTotalTorqueZ=off  CompositeWrenchDir=FollowerOnBase  CompositeWrenchFrame=BaseFrame  EquilibriumPosition=0  EquilibriumPositionUnits=deg  SpringStiffness=0  SpringStiffnessUnits=N*m/deg  DampingCoefficient=0  DampingCoefficientUnits=N*m/(deg/s)  TorqueActuationMode=NoTorque  MotionActuationMode=ComputedMotion  SensePosition=off  SenseVelocity=off  SenseAcceleration=off  SenseTorqueForce=off  PositionTargetValue=0  PositionTargetValueUnits=deg  PositionTargetSpecify=off  PositionTargetPriority=High  VelocityTargetValue=0  VelocityTargetValueUnits=deg/s  VelocityTargetSpecify=off  VelocityTargetPriority=High  BlockFunction=simmechanics.library.joints.revolute_joint
  Rotor Conn : PMIOPort  Port=1  Side=Left
  Gearhead Position [rad] : Outport
  Gearhead Velocity [rad/s] : Outport  Port=2
  Rotor Velocity [rad/s] : Outport  Port=3
  wires:
  PS-Simulink Converter1/1 -> Gearhead Position [rad]/1
  Rotor Torque [Nm]/1 -> Sum/1
  PS-Simulink Converter2/1 -> Gearhead Velocity [rad/s]/1
  PS-Simulink Converter3/1 -> Rotor Velocity [rad/s]/1
  Spring Torque [Nm]/1 -> Opposite/1
  Opposite/1 -> Simulink-PS Converter1/1
  PS-Simulink Converter/1 -> Sum/2
  Sum/1 -> Simulink-PS Converter/1
  connections:
  Virtual Gear Joint/RConn1 -- Virtual Follower Gear/RConn1 -- Virtual Gear Constraint/RConn1 -- Idler Gear Constraint/LConn1
  External Force and Torque/RConn1 -- Output Gear/RConn1 -- Aligned Gear Constraint/RConn1 -- Output Gear Joint/RConn1
  Gear Offset/RConn1 -- Virtual Gear Joint/LConn1
  Gear Offset/LConn1 -- Rotor Joint/LConn1 -- Rotor Conn/RConn1 -- Output Gear Joint/LConn1 -- Idler Offset/LConn1
  Rotor Joint/RConn1 -- Virtual Gear Constraint/LConn1 -- Rotor + Base Gear/RConn1
  Rotor Joint/LConn2 -- Simulink-PS Converter/RConn1
  PS-Simulink Converter2/LConn1 -- Output Gear Joint/RConn3
  PS-Simulink Converter1/LConn1 -- Output Gear Joint/RConn2
  PS-Simulink Converter3/LConn1 -- Rotor Joint/RConn2 -- Rotational Simscape Intf/LConn1
  Simulink-PS Converter1/RConn1 -- External Force and Torque/LConn1
  Idler Gear Constraint/RConn1 -- Virtual Idler/RConn1 -- Idler Gear/RConn1 -- Aligned Gear Constraint/LConn1
  Idler Offset/RConn1 -- Virtual Idler/LConn1
  Rotational Simscape Intf/RConn2 -- Mechanical Rotational Reference/LConn1 -- Rotational Friction/RConn1
  Rotational Friction/LConn1 -- Rotational Simscape Intf/LConn2
  PS-Simulink Converter/LConn1 -- Rotational Simscape Intf/RConn1

== system coalesce_walk_2d_sim/Mechanical Simulation Layer/Left Hip Roll Joint/Mechanical Limits /Enabled Subsystem ==
  Col_Flags : Inport
  Enable : EnablePort  StatesWhenEnabling=reset  ZeroCross=off
  To Workspace : ToWorkspace  VariableName=L_roll_collision_flags  SampleTime=-1
  wires:
  Col_Flags/1 -> To Workspace/1

== system coalesce_walk_2d_sim/Mechanical Simulation Layer/Left Hip Roll Joint/Mechanical Limits /Roll Max Collision Model ==
  note: Mechanical Limits Model
  phi [rad] : Inport
  vphi [rad/s] : Inport  Port=2
  Contact! : EnablePort  StatesWhenEnabling=reset
  Gain3 : Gain  Gain=k_phi
  Gain4 : Gain  Gain=1/v_phi_max
  Mux1 : Mux  Inputs=2
  Reaction Force : Fcn  Expr="- u(1)  *  (1-u(2)) * (u(2)<1)"
  tau_interaction[Nm] : Outport  OutputWhenDisabled=reset  InitialOutput=0
      settings: AttributesFormatString=initial = '%<InitialOutput>'\nwhen disabled = '%<OutputWhenDisabled>'
  wires:
  Reaction Force/1 -> tau_interaction[Nm]/1
  phi [rad]/1 -> Gain3/1
  vphi [rad/s]/1 -> Gain4/1
  Mux1/1 -> Reaction Force/1
  Gain3/1 -> Mux1/1
  Gain4/1 -> Mux1/2

== system coalesce_walk_2d_sim/Mechanical Simulation Layer/Left Hip Roll Joint/Mechanical Limits /Roll Min Collision Model ==
  note: Mechanical Limits Model
  phi [rad] : Inport
  vphi [rad/s] : Inport  Port=2
  Contact! : EnablePort  StatesWhenEnabling=reset
  Gain3 : Gain  Gain=k_phi
  Gain4 : Gain  Gain=1/v_phi_max
  Mux1 : Mux  Inputs=2
  Reaction Force : Fcn  Expr="- u(1)  *  (1-u(2)) * (u(2)<1)"
  tau_interaction[Nm] : Outport  OutputWhenDisabled=reset  InitialOutput=0
      settings: AttributesFormatString=initial = '%<InitialOutput>'\nwhen disabled = '%<OutputWhenDisabled>'
  wires:
  Gain4/1 -> Mux1/2
  Gain3/1 -> Mux1/1
  Mux1/1 -> Reaction Force/1
  vphi [rad/s]/1 -> Gain4/1
  phi [rad]/1 -> Gain3/1
  Reaction Force/1 -> tau_interaction[Nm]/1

== system coalesce_walk_2d_sim/Mechanical Simulation Layer/R Ground Contact/Ground Friction Model/Friction Switch ==
  note: Static/Kinetic Friction Switch
  Slide! : Inport
  Stick! : Inport  Port=2
  Memory : Memory  InheritSampleTime=on
  S-R Flip-Flop : simulink_extras/Flip Flops/S-R Flip-Flop  initial_condition=0
  Terminator : Terminator
  Stiction : Outport
  wires:
  S-R Flip-Flop/1 -> Memory/1
  S-R Flip-Flop/2 -> Terminator/1
  Stick!/1 -> S-R Flip-Flop/1
  Slide!/1 -> S-R Flip-Flop/2
  Memory/1 -> Stiction/1

== system coalesce_walk_2d_sim/Mechanical Simulation Layer/R Ground Contact/Ground Friction Model/t-Axis Kinetic Friction Model ==
  note: Kinetic Friction Model
  note: Footpoint Determiner
  note: Sliding Limit Detector
  pos_x [m] : Inport
  vel_x [m/s] : Inport  Port=2
  pos_z [m] : Inport  Port=3
  vel_z [m/s] : Inport  Port=4
  F_Normal [N] : Inport  Port=5
  Enable : EnablePort  StatesWhenEnabling=reset  ZeroCross=off
  Constant : Constant  Value=vLimit
  Constant1 : Constant  Value=eps
  Demux : Demux  Outputs=2
  Divide : Product  Inputs=*/
  FixPt Relational Operator : RelationalOperator  Operator=>  OutDataTypeStr=boolean  ZeroCross=off
  Magnitude : Subsystem
  Memory : Memory  InheritSampleTime=on
  Mux : Mux  Inputs=2
  Negative : simulink/Logic and Bit Operations/Compare To Zero  relop=<  OutDataTypeStr=boolean
  Product : Product  RndMeth=Zero
  Sum : Sum  Inputs=|+-
  Sum1 : Sum  Inputs=|++
  reverse : Gain  Gain=-1
  sliding friction coefficient : Gain  Gain=mu_slide
  posFP_x [m] : Outport  InitialOutput=0
      settings: AttributesFormatString=initial = '%<InitialOutput>'\nwhen disabled = '%<OutputWhenDisabled>'
  posFP_z [m] : Outport  Port=2  InitialOutput=0
      settings: AttributesFormatString=initial = '%<InitialOutput>'\nwhen disabled = '%<OutputWhenDisabled>'
  Stiction! : Outport  Port=3  OutputWhenDisabled=reset  InitialOutput=0
      settings: AttributesFormatString=initial = '%<InitialOutput>'\nwhen disabled = '%<OutputWhenDisabled>'
  Fx_Slide [N] : Outport  Port=4  OutputWhenDisabled=reset  InitialOutput=0
      settings: AttributesFormatString=initial = '%<InitialOutput>'\nwhen disabled = '%<OutputWhenDisabled>'
  Fz_Slide [N] : Outport  Port=5  OutputWhenDisabled=reset  InitialOutput=0
      settings: AttributesFormatString=initial = '%<InitialOutput>'\nwhen disabled = '%<OutputWhenDisabled>'
  wires:
  reverse/1 -> Product/1
  F_Normal [N]/1 -> sliding friction coefficient/1
  pos_x [m]/1 -> posFP_x [m]/1
  sliding friction coefficient/1 -> Product/2
  Divide/1 -> reverse/1
  FixPt Relational Operator/1 -> Stiction!/1
  Memory/1 -> FixPt Relational Operator/2
  Negative/1 -> Memory/1, FixPt Relational Operator/1
  Magnitude/1(Magnitude) -> Sum/1, Sum1/1
  Sum/1 -> Negative/1
  Constant/1 -> Sum/2
  pos_z [m]/1 -> posFP_z [m]/1
  vel_x [m/s]/1 -> Mux/1
  vel_z [m/s]/1 -> Mux/2
  Mux/1 -> Divide/1, Magnitude/1(Vector)
  Constant1/1 -> Sum1/2
  Sum1/1 -> Divide/2
  Product/1 -> Demux/1
  Demux/1 -> Fx_Slide [N]/1
  Demux/2 -> Fz_Slide [N]/1
